simulink model "rtwdemo_mpf"  (Simulink 7.6)
settings: Solver=FixedStepDiscrete  StartTime=0.0  StopTime=1  FixedStep=0.001  RelTol=1e-3
PostLoadFcn:
  | evalin('base','clear;');
  | F1=2;Gain1=5;Gain2=-3;G1=6;G2=-2.6;G3=9;
Description:
  | Data packaging examples
settings Model: Creator=The MathWorks Inc.  ExtModeAutoUpdateStatusClock=off
settings MATStruct: SampleTime=0.001  Offset=0  Priority=[20.0]
settings DataIOCC: SaveOutput=off  SaveTime=off
settings OptimizationCC: InlineParams=on  InlineInvariantSignals=on  PassReuseOutputArgsAs=Individual arguments  StateBitsets=on  DataBitsets=on  UseTempVars=on  ZeroExternalMemoryAtStartup=off  ZeroInternalMemoryAtStartup=off  NoFixptDivByZeroProtection=on  EfficientFloat2IntCast=on  EfficientMapNaN2IntZero=off  OptimizeModelRefInitCode=on  LifeSpan=1  BufferReusableBoundary=off
settings DebuggingCC: CheckExecutionContextPreStartOutputMsg=on  CheckExecutionContextRuntimeOutputMsg=on  SigSpecEnsureSampleTimeMsg=none  StrictBusMsg=ErrorOnBusTreatedAsVector
settings HardwareCC: ProdIntDivRoundTo=Zero  ProdEndianess=LittleEndian  ProdHWDeviceType=Generic->32-bit Embedded Processor  TargetHWDeviceType=Generic->32-bit Embedded Processor
settings SFSimCC: SimParseCustomCode=off
settings RTWCC: SystemTargetFile=ert.tlc  TemplateMakefile=ert_default_tmf  Description=RTW Embedded Coder (no auto configuration)  GenerateReport=on  RTWVerbose=off  ProcessScript=ert_make_rtw_hook  IncludeHyperlinkInReport=on  LaunchReport=on
settings CodeAppCC: ForceParamTrailComments=on  IgnoreCustomStorageClasses=off  IgnoreTestpoints=on  SimulinkDataObjDesc=on  CustomSymbolStrGlobalVar=rt$N$M  CustomSymbolStrType=$N$M  CustomSymbolStrFcn=$N$M$F  CustomSymbolStrMacro=$N$M  InsertBlockDesc=on
settings ERTTargetCC: TargetFcnLib=ansi_tfl_tmw.mat  MultiwordLength=2048  GenerateSampleERTMain=on  SupportNonFinite=off  InlinedParameterPlacement=NonHierarchical  ERTCustomFileTemplate=example_file_process.tlc  DataDefinitionFile=global  ERTFilePackagingFormat=CompactWithDataFile  DataReferenceFile=global  ConvertIfToSwitch=off

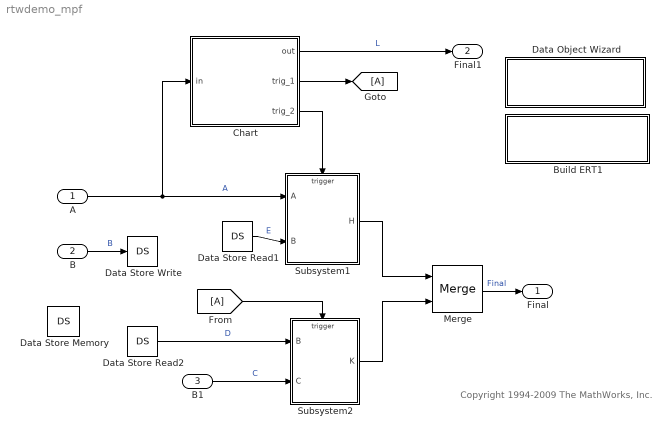
== system rtwdemo_mpf ==
  note: Copyright 1994-2009 The MathWorks, Inc.
  A : Inport  OutDataTypeStr=double  PortDimensions=1  SampleTime=0.001
  B : Inport  Port=2  OutDataTypeStr=double  PortDimensions=1  SampleTime=0.001
  B1 : Inport  Port=3  OutDataTypeStr=double  PortDimensions=1  SampleTime=0.001
  Build ERT1 : Subsystem  mask{attrib_overrides={}}
      mask prompts: attrib_overrides "List of attributes to preserve (cell of strings):"
      mask help: Invoke Model Explorer
      settings: OpenFcn=daexplr;
      mask Display:
      | disp(['Invoke Model Explorer\n',...
      | 	  '(Double click.)'])
  Chart : Stateflow chart  TreatAsAtomicUnit=on  RTWFcnName=entry_point  RTWFileName=sfcc
      settings: RTWSystemCode=Function  RTWFcnNameOpts=User specified
  Data Object Wizard : Subsystem  Description=DOW
      settings: OpenFcn=dataobjectwizard(bdroot);
      mask Type: Data Object Wizard
      mask Description: Simulink data object wizard for creating potential Simulink data objects.
      mask Help: helpview([docroot,'/toolbox/ecoder/helptargets.map'],'data_obj_wiz');
      mask Display: disp('Invoke Data\nObject Wizard\n(Double click.)');
  Data Store Memory : DataStoreMemory  DataStoreName=DS
  Data Store Read1 : DataStoreRead  DataStoreName=DS  SampleTime=0.001
  Data Store Read2 : DataStoreRead  DataStoreName=DS  SampleTime=0.001
  Data Store Write : DataStoreWrite  DataStoreName=DS
  Merge : Merge
  Subsystem1 : Subsystem
  Subsystem2 : Subsystem
  Final : Outport
  Final1 : Outport  Port=2
  wires:
  B1/1 -> Subsystem2/2(C)  "C"
  A/1 -> Subsystem1/1(A), Chart/1(in)  "A"
  Subsystem1/1(H) -> Merge/1
  Subsystem2/1(K) -> Merge/2
  Merge/1 -> Final/1  "Final"
  Chart/3(trig_2) -> Subsystem1/Trigger
  Chart/2(trig_1) -> [A]
  [A] -> Subsystem2/Trigger
  Chart/1(out) -> Final1/1  "L"
  B/1 -> Data Store Write/1  "B"
  Data Store Read1/1 -> Subsystem1/2(B)  "E"
  Data Store Read2/1 -> Subsystem2/1(B)  "D"

== system rtwdemo_mpf/Build ERT1 ==

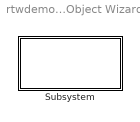
== system rtwdemo_mpf/Data Object Wizard ==
  Subsystem : Subsystem

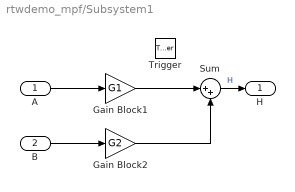
== system rtwdemo_mpf/Subsystem1 ==
  A : Inport
  B : Inport  Port=2
  Trigger : TriggerPort  TriggerType=function-call
  Gain Block1 : Gain  Gain=G1
  Gain Block2 : Gain  Gain=G2
  Sum : Sum  Inputs=|++
  H : Outport
  wires:
  A/1 -> Gain Block1/1
  Gain Block1/1 -> Sum/1
  B/1 -> Gain Block2/1
  Gain Block2/1 -> Sum/2
  Sum/1 -> H/1  "H"

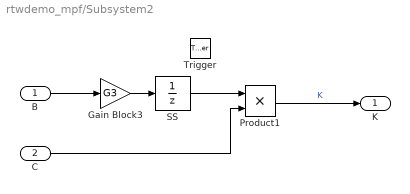
== system rtwdemo_mpf/Subsystem2 ==
  B : Inport
  C : Inport  Port=2
  Trigger : TriggerPort  TriggerType=function-call
  Gain Block3 : Gain  Gain=G3
  Product1 : Product  RndMeth=Zero
  SS : UnitDelay  SampleTime=-1  StateIdentifier=SS
  K : Outport
  wires:
  B/1 -> Gain Block3/1
  Gain Block3/1 -> SS/1
  C/1 -> Product1/2
  Product1/1 -> K/1  "K"
  SS/1 -> Product1/1

== system rtwdemo_mpf/Data Object Wizard/Subsystem ==

== stateflow chart Chart ==
  (default) -> (junction 3)
  (junction 3) -> (junction 4) [order 2] : {
      | out = in;
      | trig_2;
      | }
  (junction 3) -> (junction 4) [order 1] : [ in*F1 > 10]
      | {
      | out = in * Gain1 * Gain2;
      | trig_1;
      | }
  data: Gain1 parameter double; Gain2 parameter double; in input double; out output double; F1 parameter double
  events: trig_1 output FUNCTION_CALL_EVENT; trig_2 output FUNCTION_CALL_EVENT
